simulink model "current_filter_model"  (R2023b)
settings: Solver=FixedStepDiscrete  StartTime=0.0  StopTime=0.020  FixedStep=5e-5  RelTol=1e-3
undefined symbols (not defined in the file or in its folder): current_filter_test
settings Model: DataDictionary=current_filter_interface.sldd  Creator=user  LastModifiedBy=user
settings OptimizationCC: EnhancedBackFolding=on  PassReuseOutputArgsAs=Individual arguments  OptimizeBlockOrder=speed  DifferentSizesBufferReuse=on  OptimizationCustomize=off  EfficientTunableParamExpr=on
settings DebuggingCC: ParameterTunabilityLossMsg=error
settings SFSimCC: MATLABDynamicMemAlloc=off
settings RTWCC: Description=Embedded Coder  SystemTargetFile=ert.tlc  GenCodeOnly=on  TemplateMakefile=ert_default_tmf  GenerateReport=on
settings CodeAppCC: ForceParamTrailComments=on  IgnoreCustomStorageClasses=off  OperatorAnnotations=on  SimulinkDataObjDesc=on  SFDataObjDesc=on  InsertBlockDesc=on
settings ERTTargetCC: TargetLangStandard=C99 (ISO)  CodeInterfacePackaging=Reusable function  ERTCustomFileTemplate=example_file_process.tlc

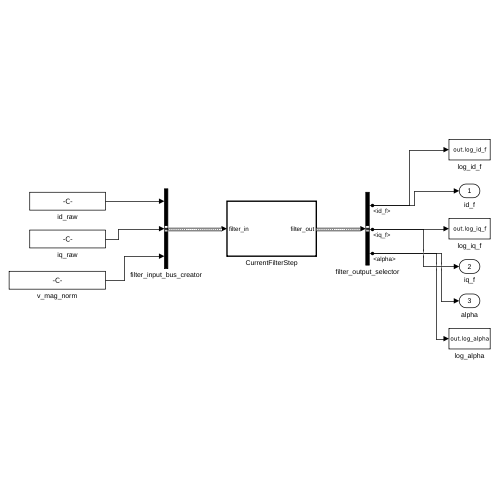
[thumbnail: Simulink's stored preview of the top-level diagram]
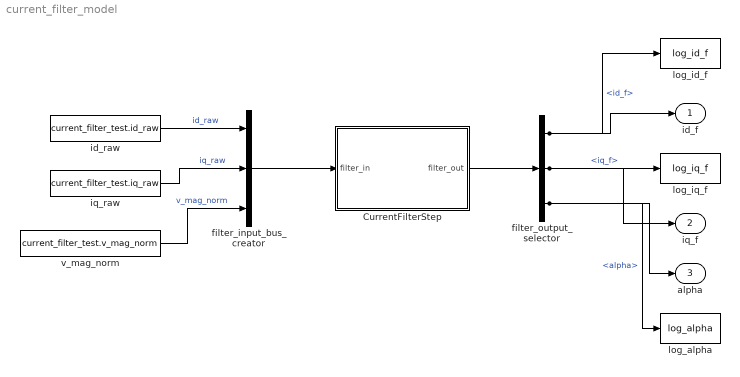
== system current_filter_model ==
  CurrentFilterStep : Subsystem  TreatAsAtomicUnit=on  RTWFcnName=CurrentFilterStep  RTWFileName=CurrentFilterStep
      settings: RTWFcnNameOpts=User specified  RTWFileNameOpts=User specified
  filter_input_bus_creator : BusCreator  Inputs=3  OutDataTypeStr=Bus: current_filter_input_t  NonVirtualBus=on
  filter_output_selector : BusSelector  OutputSignals=id_f,iq_f,alpha
  id_raw : Constant  Value=current_filter_test.id_raw  OutDataTypeStr=T_CurrentFilterCurrent  SampleTime=5e-5
  iq_raw : Constant  Value=current_filter_test.iq_raw  OutDataTypeStr=T_CurrentFilterCurrent  SampleTime=5e-5
  log_alpha : ToWorkspace  VariableName=log_alpha  SaveFormat=Structure With Time  SampleTime=-1
  log_id_f : ToWorkspace  VariableName=log_id_f  SaveFormat=Structure With Time  SampleTime=-1
  log_iq_f : ToWorkspace  VariableName=log_iq_f  SaveFormat=Structure With Time  SampleTime=-1
  v_mag_norm : Constant  Value=current_filter_test.v_mag_norm  OutDataTypeStr=T_CurrentFilterReal  SampleTime=5e-5
  id_f : Outport
  iq_f : Outport  Port=2
  alpha : Outport  Port=3
  wires:
  filter_output_selector/3 -> alpha/1, log_alpha/1  "<alpha>"
  filter_input_bus_creator/1 -> CurrentFilterStep/1(filter_in)
  filter_output_selector/2 -> iq_f/1, log_iq_f/1  "<iq_f>"
  CurrentFilterStep/1(filter_out) -> filter_output_selector/1
  v_mag_norm/1 -> filter_input_bus_creator/3  "v_mag_norm"
  filter_output_selector/1 -> id_f/1, log_id_f/1  "<id_f>"
  iq_raw/1 -> filter_input_bus_creator/2  "iq_raw"
  id_raw/1 -> filter_input_bus_creator/1  "id_raw"

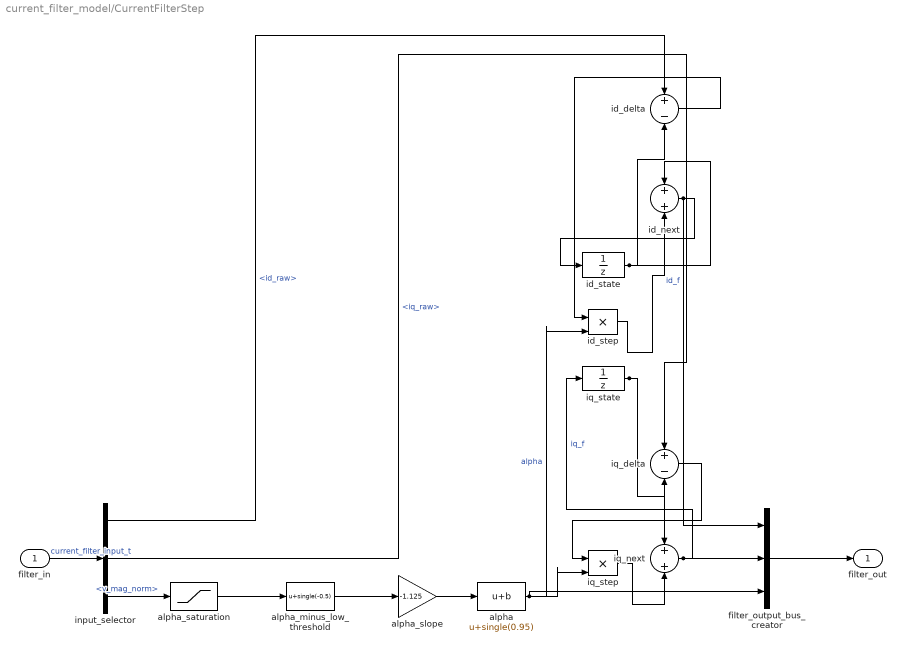
== system current_filter_model/CurrentFilterStep ==
  filter_in : Inport  OutDataTypeStr=Bus: current_filter_input_t  BusOutputAsStruct=on
  alpha : Bias  Bias=single(0.95)  SaturateOnIntegerOverflow=off
  alpha_minus_low_threshold : Bias  Bias=single(-0.5)  SaturateOnIntegerOverflow=off
  alpha_saturation : Saturate  UpperLimit=single(0.9)  LowerLimit=single(0.5)
  alpha_slope : Gain  Gain=-1.125  ParamDataTypeStr=T_CurrentFilterReal
  filter_output_bus_creator : BusCreator  Inputs=3  OutDataTypeStr=Bus: current_filter_output_t  NonVirtualBus=on
  id_delta : Sum  Inputs=+-
  id_next : Sum
  id_state : UnitDelay  SampleTime=-1  HasFrameUpgradeWarning=on
  id_step : Product
  input_selector : BusSelector  OutputSignals=id_raw,iq_raw,v_mag_norm
  iq_delta : Sum  Inputs=+-
  iq_next : Sum
  iq_state : UnitDelay  SampleTime=-1  HasFrameUpgradeWarning=on
  iq_step : Product
  filter_out : Outport  OutDataTypeStr=Bus: current_filter_output_t
  wires:
  iq_next/1 -> filter_output_bus_creator/2, iq_state/1  "iq_f"
  iq_delta/1 -> iq_step/1
  filter_in/1 -> input_selector/1  "current_filter_input_t"
  filter_output_bus_creator/1 -> filter_out/1
  input_selector/1 -> id_delta/1  "<id_raw>"
  alpha_minus_low_threshold/1 -> alpha_slope/1
  id_next/1 -> filter_output_bus_creator/1, id_state/1  "id_f"
  input_selector/2 -> iq_delta/1  "<iq_raw>"
  alpha/1 -> iq_step/2, id_step/2, filter_output_bus_creator/3  "alpha"
  input_selector/3 -> alpha_saturation/1  "<v_mag_norm>"
  alpha_slope/1 -> alpha/1
  id_step/1 -> id_next/2
  iq_state/1 -> iq_next/1, iq_delta/2
  id_state/1 -> id_next/1, id_delta/2
  alpha_saturation/1 -> alpha_minus_low_threshold/1
  iq_step/1 -> iq_next/2
  id_delta/1 -> id_step/1
